simulink model "PBMAmodel"  (R2014a)
settings: Solver=FixedStepDiscrete  StartTime=0.0  StopTime=8000  RelTol=1e-3
undefined symbols (not defined in the file): pbma_model1
libraries: identextras x30, simulink x16
(part 1 of 3)
settings Model: Creator=md596  LastModifiedBy=md596

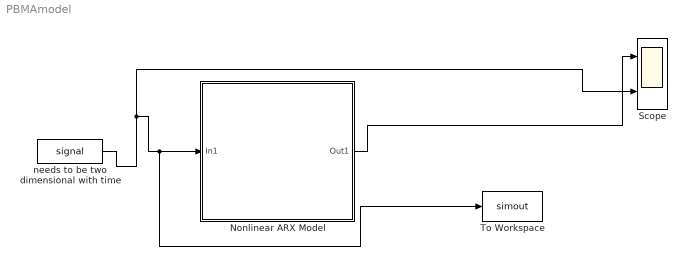
== system PBMAmodel ==
  Nonlinear ARX Model : Subsystem  AncestorBlock=slident/Models/Nonlinear ARX Model  mask(Nonlinear ARX Model){sys=pbma_model1, ICspec=Input and output values, X0=0, U0=0, Y0=0}
      mask prompts: sys "Model"; ICspec "Initial conditions:"; X0 "Specify initial states as a vector of 32 values."; U0 "Input level (scalar)"; Y0 "Output levels (scalar or vector of length equal to number of model outputs)"
      mask help:
      | Simulate a nonlinear ARX (idnlarx) model. Specify the name of an estimated idnlarx model for "Model". Specify initial conditions for simulation as one of the following:
      | 1. Steady-state (equilibrium) input and output signal levels.
      | 2. An initial state vector. Click on Help button for information on how to determine initial states from various requirements.
      mask init:
      | MaskVal = get_param(gcb,'MaskValues');
      | sysname = MaskVal{1};
      | if isa(sys,'idnlarx')
      |    maskEn = get_param(gcb,'MaskEnables');
      |    nu = size(sys,'nu');
      |    fInp = find_system(gcb,'FollowLinks','on','LookUnderMasks','all',...
      |       'SearchDepth',1,'Name','In1');
      |    
      |    if nu>0 && isempty(fInp)
      |       add_block('built-in/Inport',[gcb,'/In1'],'Position',[20   133    50   147])
      |    elseif nu==0 && ~isempty(fInp)
      |       delete_block(fInp);
      |    end
      |    %{
      |     if nu==0
      |         maskEn{4} = 'off';
      |     else
      |         maskEn{4} = 'on';
      |     end
      |    %}
      |    
      |    set_param(gcb,'MaskEnables',maskEn);
      |    
      | else
      |    sysname = '???';
      |    sys = [];
      |    U0 = [];
      |    Y0 = [];
      |    X0 = [];
      |    Nx = 0;   
      | end
      | 
      | if any(strcmp(get_param(bdroot(gcb),'SimulationStatus'),{'initializing','updating'}))
      |    lwarn = lastwarn;warn = warning('off');
      |    try
      |       [X0,Ts,WarnMsg] = idnlarxmaskinit('initialization',gcb,sys,ICspec,X0,U0,Y0);
      |       Nx = length(X0);
      |       warning(warn);lastwarn(lwarn);
      |       for i = 1:size(WarnMsg,1)
      |          warning(WarnMsg{i,1},WarnMsg{i,2})
      |       end
      |    catch E
      |       sys = [];
      |       U0 = [];
      |       Y0 = [];
      |       sysname = '???';
      |       X0 = [];
      |       Nx = 0;
      |       warning(warn);lastwarn(lwarn);
      |       throw(E)
      |    end
      | end
      mask Help: eval('identhelp(''idnlarx_block'')')
      mask Callback sys: idnlarxmaskinit('maskparamcallback',gcb)
      mask TypeOptions ICspec: Input and output values | State values
      mask Callback ICspec:
      | maskStr = get_param(gcb,'MaskValues');
      | if strcmp(maskStr{2}(1),'S')
      |     % "State values" option
      |     set_param(gcb,  'MaskVisibilities',   {'on';'on';'on';'off';'off'});
      |     %set_param(gcb,  'MaskEnables',        {'on';'on';'on';'off';'off'});
      | elseif strcmp(maskStr{2}(1),'I')
      |     % "Input and output values" option (default)
      |     set_param(gcb,  'MaskVisibilities',   {'on';'on';'off';'on';'on'});
      |     %set_param(gcb,  'MaskEnables',        {'on';'on';'off';'on';'on'});
      | end
      mask Display:
      | if strcmp(bdroot(gcb),'slident')
      |    disp('IDNLARX MODEL')
      | else
      |    disp(sysname)
      | end
  Scope : Scope  NumInputPorts=2
      settings: YMin=-5~-5  YMax=5~5
  To Workspace : ToWorkspace  VariableName=simout  SaveFormat=Timeseries  SampleTime=-1
  needs to be two dimensional with time : FromWorkspace  VariableName=signal  SampleTime=0
  wires:
  Nonlinear ARX Model/1(Out1) -> Scope/1
  needs to be two dimensional with time/1 -> Scope/2, To Workspace/1, Nonlinear ARX Model/1(In1)
